simulink model "SNAP_DETUMBLE_barbalatLemma"  (R2024a)
settings: Solver=ode45  StartTime=0.0  StopTime=SNAP_sim_length  FixedStep=0.1  MaxStep=10  MinStep=0.01  RelTol=1e-2  EnableMultiTasking=on
InitFcn:
  | SNAP_Simulink_Init_Function
values from neighbouring files (symbols this model uses):
  bias = [28.8675 28.8675 28.8675]    [SNAP_Simulink_Init_Function.m]    (also in Script_magnetorquer_and_magnetometer.m; SnapParameters.m)
  boira_Imax = boira_max_magnetic_torque./boira_magnetic_gains    [SNAP_Simulink_Init_Function.m]    (also in Script_magnetorquer_and_magnetometer.m; SnapParameters.m)
  boira_magnetic_gains = [2.3 2.3 2.1]    [SNAP_Simulink_Init_Function.m]    (also in Script_magnetorquer_and_magnetometer.m; SnapParameters.m)
  day = C - E + F - floor(30.6001 * G)    [julian2datetime.m]
  EN_2BodyModel = 1    [SNAP_Simulink_Init_Function.m]
  EN_Aero = SNAP_sim_params.aero_enabled    [SNAP_Simulink_Init_Function.m]
  EN_GG = 1    [SNAP_Simulink_Init_Function.m]
  EN_Hyst = 0    [SNAP_Simulink_Init_Function.m]
  EN_Mag = 1    [SNAP_Simulink_Init_Function.m]
  initial_position = SNAP_sim_params.initial_position    [SNAP_Simulink_Init_Function.m]
  initial_velocity = SNAP_sim_params.initial_velocity    [SNAP_Simulink_Init_Function.m]
  lookup_breakpoints_mmeter = linspace(-200,200,50)*10^3    [SNAP_Simulink_Init_Function.m]    (also in Script_magnetorquer_and_magnetometer.m; SnapParameters.m)
  lookup_breakpoints_mtorquer = linspace(-boira_Imax(1)*2,boira_Imax(1)*2,55)    [SNAP_Simulink_Init_Function.m]    (also in Script_magnetorquer_and_magnetometer.m; SnapParameters.m)
  lookup_tabledata_mmeter = lookup_breakpoints_mmeter+max_deviation_mmeter*sin(pi*lookup_breakpoints_mmeter/max_breakpoint_mmeter)    [SNAP_Simulink_Init_Function.m]    (also in Script_magnetorquer_and_magnetometer.m; SnapParameters.m)
  lookup_tabledata_mtorquer = lookup_breakpoints_mtorquer+max_deviation_mtorquer*sin(pi*lookup_breakpoints_mtorquer/max_breakpoint_mtorquer)    [SNAP_Simulink_Init_Function.m]    (also in Script_magnetorquer_and_magnetometer.m; SnapParameters.m)
  noise = 0    [SNAP_Simulink_Init_Function.m]    (also in Script_magnetorquer_and_magnetometer.m; SnapParameters.m)
  noise_variance = 30    [SNAP_Simulink_Init_Function.m]    (also in Script_magnetorquer_and_magnetometer.m; SnapParameters.m)
  rotm_mmeter = eul2rotm([missalingment_x_mmeter missalingment_y_mmeter missalingment_z_mmeter])    [SNAP_Simulink_Init_Function.m]    (also in Script_magnetorquer_and_magnetometer.m; SnapParameters.m)
  rotm_mtorquer = eul2rotm([missalingment_x_mtorquer missalingment_y_mtorquer missalingment_z_mtorquer])    [SNAP_Simulink_Init_Function.m]    (also in Script_magnetorquer_and_magnetometer.m; SnapParameters.m)
  second = (day_fraction - hour - minute / 60) * 3600    [julian2datetime.m]
  SNAP_Br = SNAP_sim_params.Br    [SNAP_Simulink_Init_Function.m]
  SNAP_Bs = SNAP_sim_params.Bs    [SNAP_Simulink_Init_Function.m]
  SNAP_CONST_a3H0 = 7.943e15    (= 7.943e+15)    [SNAP_Simulink_Init_Function.m]
  SNAP_CONST_earth_mag_dipole = [sin(168.6*pi/180)* cos(109.3*pi/180), sin(168.6*pi/180)* sin(109.3*pi/180), cos(168.6*pi/180)]    [SNAP_Simulink_Init_Function.m]
  SNAP_CONST_G_earth = 6.6742e-11    [SNAP_Simulink_Init_Function.m]
  SNAP_CONST_m_earth = 5.9736e24    (= 5.9736e+24)    [SNAP_Simulink_Init_Function.m]
  SNAP_CONST_mu0 = 4*pi*1e-7    (= 1.25663706144e-06)    [SNAP_Simulink_Init_Function.m]
  SNAP_CONST_r_earth = 6.36101e6    (= 6361010)    [SNAP_Simulink_Init_Function.m]
  SNAP_Hc = SNAP_sim_params.Hc    [SNAP_Simulink_Init_Function.m]
  SNAP_init_rates = SNAP_sim_params.init_rates    [SNAP_Simulink_Init_Function.m]
  SNAP_JD = SNAP_sim_params.JD    [SNAP_Simulink_Init_Function.m]
  SNAP_sat_inertia = boira_inertia    [SNAP_Simulink_Init_Function.m]
  SNAP_sat_mass = boira_mass    (= 2)    [SNAP_Simulink_Init_Function.m]
  SNAP_starting_ECI2ECEF_dcm = dcmeci2ecef('IAU-2000/2006',SNAP_sim_params.DateVector)    [SNAP_Simulink_Init_Function.m]
  SNAP_V_hyst = boira_V_hyst    [SNAP_Simulink_Init_Function.m]
undefined symbols (not defined in the file or in its folder): aeroCIP2006, magnitude, SNAPaero
libraries: vrlib x23, simulink x10, sharedtransform x9, aerolibutil x6, aerolibconvert2 x5, aerolibobsolete x1, aerolibanim x1, matrix_library x1
(part 1 of 2)
settings Model: PacingRate=0.010000  Creator=Samir Rawashdeh  LastModifiedBy=pimpao
settings SolverCC: AlgebraicLoopSolver=TrustRegion
settings DataIOCC: SaveFormat=Array  SignalLoggingSaveFormat=ModelDataLogs  ReturnWorkspaceOutputs=off
settings OptimizationCC: ExpressionDepthLimit=2147483647  LifeSpan=inf
settings DebuggingCC: UnderspecifiedInitializationDetection=Classic  MergeDetectMultiDrivingBlocksExec=none  SolverPrmCheckMsg=warning  MultiTaskCondExecSysMsg=warning  MultiTaskRateTransMsg=warning  SingleTaskRateTransMsg=warning  FcnCallInpInsideContextMsg=warning  UnconnectedInputMsg=warning  UnconnectedOutputMsg=warning  UnconnectedLineMsg=warning  StateNameClashWarn=warning  SFUnexpectedBacktrackingDiag=warning  SFNoUnconditionalDefaultTransitionDiag=warning  ArithmeticOperatorsInVariantConditions=warning
settings HardwareCC: ProdBitPerPointer=32  ProdBitPerSizeT=32  ProdBitPerPtrDiffT=32  ProdLargestAtomicFloat=None  ProdIntDivRoundTo=Undefined  ProdEndianess=Unspecified  ProdWordSize=32  ProdHWDeviceType=32-bit Generic
settings ModelReferenceCC: EnableRefExpFcnMdlSchedulingChecks=on  PropagateSignalLabelsOutOfModel=off
settings SFSimCC: SimUseLocalCustomCode=off  CustomCodeUndefinedFunction=UseInterfaceOnly
settings RTWCC: RTWUseLocalCustomCode=off  GPUComputeCapability=3.5
settings CodeAppCC: StateflowObjectComments=on
settings GRTTargetCC: TargetLangStandard=C89/C90 (ANSI)  CombineOutputUpdateFcns=off  GRTInterface=on
settings ConfigComp: CovMetricSettings=dw  CovSaveCumulativeToWorkspaceVar=on  CovSaveSingleToWorkspaceVar=on  CovExternalEMLEnable=off  CovSFcnEnable=off

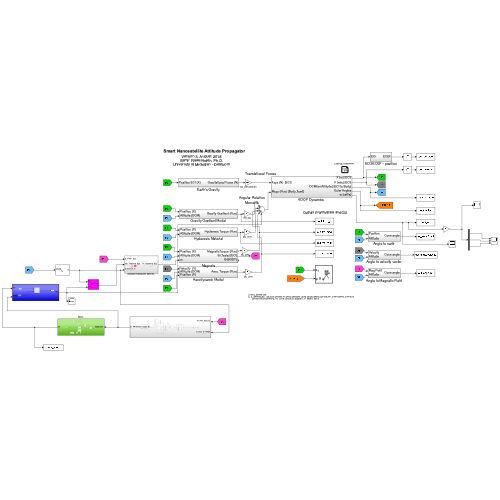
[thumbnail: Simulink's stored preview of the top-level diagram]
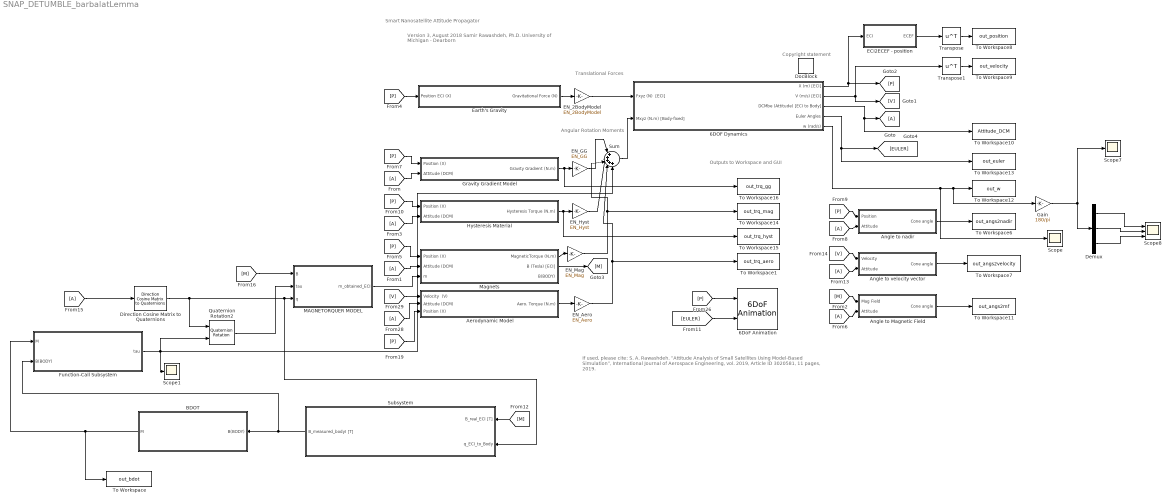
== system SNAP_DETUMBLE_barbalatLemma ==
  note: If used, please cite:
      | S. A. Rawashdeh. “Attitude Analysis of Small Satellites Using Model-Based Simulation”, International Journal of
      |       Aerospace Engineering, vol. 2019, Article ID 3020581, 11 pages, 2019.
  note: Copyright statement
  note: Smart Nanosatellite Attitude Propagator
  note: Version 3, August 2018
      | Samir Rawashdeh, Ph.D.
      | University of Michigan - Dearborn
  note: Translational Forces
  note: Angular Rotation
      | Moments
  note: Outputs to Workspace and GUI
  "6DOF Dynamics " : Subsystem
  6DoF Animation : aerolibanim/6DoF Animation  u1=[-4000 4000 -2000 2000 -5000 -3000]  u2=10  u3=1000000*4  u4=[0 0 0]  u5=Fixed position  u6=[ 1 1 1 ] * 40000000  u7=15  u8=on
  Aerodynamic Model : Subsystem
  Angle to Magnetic Field : Subsystem
  Angle to nadir : Subsystem
  Angle to velocity vector : Subsystem
  BDOT : Subsystem
  Demux : Demux  Outputs=3
  Direction Cosine Matrix to Quaternions : sharedtransform/Direction Cosine Matrix  to Quaternions  aMode=0  action=None  tolerance=eps(2)
      settings: LibrarySourceBlock=|
      | aerolibtransform2/Direction Cosine Matrix
      | to Quaternions
  DocBlock : simulink/Model-Wide Utilities/DocBlock  DocumentType=Text
      content=|
      | % See "help.txt" for documentation. More info in can be found at:
      | % sar-lab.net/snap
      | %
      | % -----------------------------------------------------------------------------
      | %   Copyright (c) 2010-2018 Samir A. Rawashdeh
      | %   Electrical and Computer Engineering
      | %   University of Michigan - Dearborn
      | %
      | %   All rights reserved.
      | %
      | %   Redistribution and use in source and binary forms, with or without
      | %   modification, are permitted provided that the following conditions are
      | %   met:
      | %
      | %       * Redistributions of source code must retain the above copyright
      | %         notice, this list of conditions and the following disclaimer.
      | %       * Redistributions in binary form must reproduce the above copyright
      | %         notice, this list of conditions and the following disclaimer in
      | %         the documentation and/or other materials provided with the distribution
      | %
      | %   THIS SOFTWARE IS PROVIDED BY THE COPYRIGHT HOLDERS AND CONTRIBUTORS "AS IS"
      | %   AND ANY EXPRESS OR IMPLIED WARRANTIES, INCLUDING, BUT NOT LIMITED TO, THE
      | %   IMPLIED WARRANTIES OF MERCHANTABILITY AND FITNESS FOR A PARTICULAR PURPOSE
      | %   ARE DISCLAIMED. IN NO EVENT SHALL THE COPYRIGHT OWNER OR CONTRIBUTORS BE
      | %   LIABLE FOR ANY DIRECT, INDIRECT, INCIDENTAL, SPECIAL, EXEMPLARY, OR
      | %   CONSEQUENTIAL DAMAGES (INCLUDING, BUT NOT LIMITED TO, PROCUREMENT OF
      | %   SUBSTITUTE GOODS OR SERVICES; LOSS OF USE, DATA, OR PROFITS; OR BUSINESS
      | %   INTERRUPTION) HOWEVER CAUSED AND ON ANY THEORY OF LIABILITY, WHETHER IN
      | %   CONTRACT, STRICT LIABILITY, OR TORT (INCLUDING NEGLIGENCE OR OTHERWISE)
      | %   ARISING IN ANY WAY OUT OF THE USE OF THIS SOFTWARE, EVEN IF ADVISED OF THE
      | %   POSSIBILITY OF SUCH DAMAGE.
      | %
      | % ----------------------------------------------------------------------------
  ECI2ECEF - position : Subsystem
  EN_2BodyModel : Gain  Gain=EN_2BodyModel
  "EN_Aero " : Gain  Gain=EN_Aero
  EN_GG : Gain  Gain=EN_GG
  EN_Hyst : Gain  Gain=EN_Hyst
  EN_Mag : Gain  Gain=EN_Mag
  Earth's Gravity : Subsystem
  From{,1,3,6,8,13,15,28} (8 alike) : From
      From settings: CloseFcn=tagdialog Close
      From1 settings: CloseFcn=tagdialog Close
      From13 settings: CloseFcn=tagdialog Close
      From28 settings: CloseFcn=tagdialog Close
      From3 settings: CloseFcn=tagdialog Close
      From6 settings: CloseFcn=tagdialog Close
      From8 settings: CloseFcn=tagdialog Close
  Function-Call Subsystem : Subsystem  TreatAsAtomicUnit=on
  Gain : Gain  Gain=180/pi
  Goto : Goto
  Gravity Gradient Model : Subsystem
  Hysteresis Material : Subsystem
  MAGNETORQUER MODEL : Subsystem
  Magnets : Subsystem
  Quaternion Rotation2 : aerolibutil/Quaternion Rotation
  Scope : Scope
  Scope1 : Scope
  Scope7 : Scope
  Scope8 : Scope  NumInputPorts=3
  Subsystem : Subsystem
  Sum : Sum  Inputs=|+++++
  To Workspace : ToWorkspace  VariableName=out_bdot  SaveFormat=Structure With Time  SampleTime=-1
  To Workspace1 : ToWorkspace  VariableName=out_trq_aero  SaveFormat=Structure With Time  SampleTime=-1
  To Workspace10 : ToWorkspace  VariableName=Attitude_DCM  SaveFormat=Structure With Time  SampleTime=-1
  To Workspace11 : ToWorkspace  VariableName=out_angs2mf  SaveFormat=Structure With Time  SampleTime=-1
  To Workspace12 : ToWorkspace  VariableName=out_w  SaveFormat=Structure With Time  SampleTime=-1
  To Workspace13 : ToWorkspace  VariableName=out_euler  SaveFormat=Structure With Time  SampleTime=-1
  To Workspace14 : ToWorkspace  VariableName=out_trq_mag  SaveFormat=Structure With Time  SampleTime=-1
  To Workspace15 : ToWorkspace  VariableName=out_trq_hyst  SaveFormat=Structure With Time  SampleTime=-1
  To Workspace16 : ToWorkspace  VariableName=out_trq_gg  SaveFormat=Structure With Time  SampleTime=-1
  To Workspace6 : ToWorkspace  VariableName=out_angs2nadir  SaveFormat=Structure With Time  SampleTime=-1
  To Workspace7 : ToWorkspace  VariableName=out_angs2velocity  SaveFormat=Structure With Time  SampleTime=-1
  To Workspace8 : ToWorkspace  VariableName=out_position  SaveFormat=Structure With Time  SampleTime=-1
  To Workspace9 : ToWorkspace  VariableName=out_velocity  SaveFormat=Structure With Time  SampleTime=-1
  Transpose : Math  Operator=transpose  SignedPower=on
  Transpose1 : Math  Operator=transpose  SignedPower=on
  wires:
  Transpose/1 -> To Workspace8/1
  Transpose1/1 -> To Workspace9/1
  "6DOF Dynamics "/3(DCMbe (Attitude) [ECI to Body]) -> To Workspace10/1, Goto/1
  "6DOF Dynamics "/4(Euler Angles) -> [EULER], To Workspace13/1
  "6DOF Dynamics "/5(w (rad/s)) -> Scope/1, Gain/1, To Workspace12/1
  Gravity Gradient Model/1(Gravity Gradient (N.m)) -> To Workspace16/1, EN_GG/1
  Hysteresis Material/1(Hysteresis Torque (N.m)) -> EN_Hyst/1, To Workspace15/1
  EN_Mag/1 -> Sum/3, To Workspace14/1
  Angle to nadir/1(Cone angle) -> To Workspace6/1
  Angle to velocity vector/1(Cone angle) -> To Workspace7/1
  [P] -> Earth's Gravity/1(Position ECI (X))
  "6DOF Dynamics "/1(X (m) [ECI]) -> ECI2ECEF - position/1(ECI), [P]
  "6DOF Dynamics "/2(V (m/s) [ECI]) -> Transpose1/1, [V]
  [P] -> Gravity Gradient Model/1(Position (X))
  From/1 -> Gravity Gradient Model/2(Attitude (DCM))
  [P] -> Magnets/1(Position (X))
  From1/1 -> Magnets/2(Attitude (DCM))
  Magnets/1(MagneticTorque (N.m)) -> EN_Mag/1
  From8/1 -> Angle to nadir/2(Attitude)
  [P] -> Angle to nadir/1(Position)
  From13/1 -> Angle to velocity vector/2(Attitude)
  [V] -> Angle to velocity vector/1(Velocity)
  ECI2ECEF - position/1(ECEF) -> Transpose/1
  Magnets/2(B (Tesla) [ECI]) -> [M]
  Earth's Gravity/1(Gravitational Force (N)) -> EN_2BodyModel/1
  From6/1 -> Angle to Magnetic Field/2(Attitude)
  Angle to Magnetic Field/1(Cone angle) -> To Workspace11/1
  [M] -> Angle to Magnetic Field/1(Mag Field)
  EN_GG/1 -> Sum/1
  EN_Hyst/1 -> Sum/2
  [V] -> Aerodynamic Model/1(Velocity  (V))
  From28/1 -> Aerodynamic Model/2(Attitude (DCM))
  [P] -> Aerodynamic Model/3(Position (X))
  [P] -> 6DoF Animation/1
  EN_2BodyModel/1 -> "6DOF Dynamics "/1(Fxyz (N)  [ECI])
  Sum/1 -> "6DOF Dynamics "/2(Mxyz (N.m) [Body-fixed])
  [P] -> Hysteresis Material/1(Position (X))
  From3/1 -> Hysteresis Material/2(Attitude (DCM))
  Aerodynamic Model/1(Aero. Torque (N.m)) -> "EN_Aero "/1
  "EN_Aero "/1 -> Sum/4, To Workspace1/1
  [EULER] -> 6DoF Animation/2
  Gain/1 -> Scope7/1, Demux/1
  Demux/1 -> Scope8/1
  Demux/2 -> Scope8/2
  Demux/3 -> Scope8/3
  MAGNETORQUER MODEL/1(m_obtained_ECI) -> Magnets/3(m)
  Direction Cosine Matrix to Quaternions/1 -> Quaternion Rotation2/1, MAGNETORQUER MODEL/3(q), Subsystem/2(q_ECI_to_Body)
  [M] -> MAGNETORQUER MODEL/1(B)
  Function-Call Subsystem/1(tau) -> Quaternion Rotation2/2, Sum/5, Scope1/1
  Quaternion Rotation2/1 -> MAGNETORQUER MODEL/2(tau)
  BDOT/1(M) -> To Workspace/1, Function-Call Subsystem/1(M)
  Subsystem/1(B_measured_bodyI [T]) -> Function-Call Subsystem/2(B(BODY)), BDOT/1(B(BODY))
  [M] -> Subsystem/1(B_real_ECI [T])
  From15/1 -> Direction Cosine Matrix to Quaternions/1

== system SNAP_DETUMBLE_barbalatLemma/6DOF Dynamics  ==
  Fxyz (N)  [ECI] : Inport
  Mxyz (N.m) [Body-fixed] : Inport  Port=2
  Rotations - 6DoF (Quaternion) : aerolibobsolete/6DoF (Euler Angles)  units=Metric (MKS)  mtype=Fixed  rep=Quaternion  xme_0=[0 0 0] % not used  Vm_0=[0 0 0] % not used  eul_0=[0 0 0] %[0 pi/1.1 0]  pm_0=SNAP_init_rates %(ones(1,3)*0.5-rand(1,3) )* 2 * .3 *pi/180;  mass_0=SNAP_sat_mass  mass_e=0  mass_f=0  inertia=SNAP_sat_inertia  inertia_e=eye(3)  inertia_f=eye(3)  k_quat=1.0
  Terminator{,1..3,5} (5 alike) : Terminator
  Translation : Subsystem
  zero : Constant  Value=[0 0 0]
  X (m) [ECI] : Outport
  V (m/s) [ECI] : Outport  Port=2
  DCMbe (Attitude) [ECI to Body] : Outport  Port=3
  Euler Angles : Outport  Port=4
  w (rad/s) : Outport  Port=5
  wires:
  Rotations - 6DoF (Quaternion)/2 -> Terminator/1
  Rotations - 6DoF (Quaternion)/1 -> Terminator2/1
  Rotations - 6DoF (Quaternion)/5 -> Terminator1/1
  Translation/1(Xe(m) (ECI)) -> X (m) [ECI]/1
  Translation/2(Ve(m/s) (ECI)) -> V (m/s) [ECI]/1
  Rotations - 6DoF (Quaternion)/6 -> w (rad/s)/1
  Rotations - 6DoF (Quaternion)/8 -> Terminator5/1
  Rotations - 6DoF (Quaternion)/7 -> Terminator3/1
  zero/1 -> Rotations - 6DoF (Quaternion)/1
  Fxyz (N)  [ECI]/1 -> Translation/1(Fxyz (N) (inECI))
  Mxyz (N.m) [Body-fixed]/1 -> Rotations - 6DoF (Quaternion)/2
  Rotations - 6DoF (Quaternion)/3 -> Euler Angles/1
  Rotations - 6DoF (Quaternion)/4 -> DCMbe (Attitude) [ECI to Body]/1

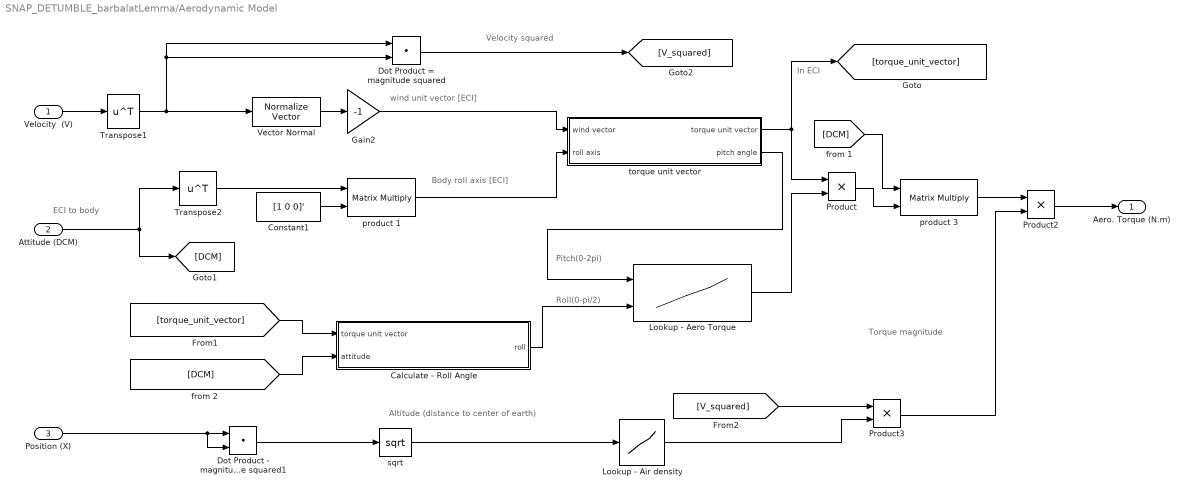
== system SNAP_DETUMBLE_barbalatLemma/Aerodynamic Model ==
  note: Pitch(0-2pi)
  note: wind unit vector [ECI]
  note: Torque magnitude
  note: Body roll axis [ECI]
  note: In ECI
  note: ECI to body
  note: Velocity squared
  note: Roll(0-pi/2)
  note: Altitude (distance to center of earth)
  Velocity  (V) : Inport
  Attitude (DCM) : Inport  Port=2
  Position (X) : Inport  Port=3
  Calculate - Roll Angle : Subsystem
  Constant1 : Constant  Value=[1 0 0]'
  Dot Product - magnitude squared1 : DotProduct  OutDataTypeStr=Inherit: Inherit via internal rule
  Dot Product = magnitude squared : DotProduct  OutDataTypeStr=Inherit: Inherit via internal rule
  Gain2 : Gain  Gain=-1
  Lookup - Aero Torque : Lookup2D  RowIndex=SNAPaero.pitch  ColumnIndex=SNAPaero.roll  Table=SNAPaero.T  SaturateOnIntegerOverflow=off  InputSameDT=off
  Lookup - Air density : Lookup  InputValues=SNAPaero.alt_range*1000 + SNAP_CONST_r_earth  Table=SNAPaero.av_density_vs_alt  SaturateOnIntegerOverflow=off
  Product : Product  RndMeth=Zero
  Product2 : Product  RndMeth=Zero
  Product3 : Product  RndMeth=Zero
  Transpose1 : Math  Operator=transpose  SignedPower=on
  Transpose2 : Math  Operator=transpose  SignedPower=on
  Vector Normal : vrlib/Utilities/Normalize Vector  maxzero=0
  product 1 : Product  Multiplication=Matrix(*)  RndMeth=Zero
  product 3 : Product  Multiplication=Matrix(*)  RndMeth=Zero
  sqrt : Math  Operator=sqrt  SignedPower=on
  torque unit vector : Subsystem
  Aero. Torque (N.m) : Outport
  wires:
  Velocity  (V)/1 -> Transpose1/1
  Dot Product = magnitude squared/1 -> [V_squared]
  Vector Normal/1 -> Gain2/1
  Gain2/1 -> torque unit vector/1(wind vector)
  product 1/1 -> torque unit vector/2(roll axis)
  torque unit vector/1(torque unit vector) -> Product/1, [torque_unit_vector]
  Lookup - Aero Torque/1 -> Product/2
  [DCM] -> product 3/1
  Transpose1/1 -> Vector Normal/1, Dot Product = magnitude squared/2, Dot Product = magnitude squared/1
  Constant1/1 -> product 1/2
  Attitude (DCM)/1 -> [DCM], Transpose2/1
  Product/1 -> product 3/2
  Calculate - Roll Angle/1(roll) -> Lookup - Aero Torque/2
  torque unit vector/2(pitch angle) -> Lookup - Aero Torque/1
  Transpose2/1 -> product 1/1
  [torque_unit_vector] -> Calculate - Roll Angle/1(torque unit vector)
  [DCM] -> Calculate - Roll Angle/2(attitude)
  Position (X)/1 -> Dot Product - magnitude squared1/1, Dot Product - magnitude squared1/2
  Dot Product - magnitude squared1/1 -> sqrt/1
  sqrt/1 -> Lookup - Air density/1
  Lookup - Air density/1 -> Product3/2
  Product3/1 -> Product2/2
  [V_squared] -> Product3/1
  Product2/1 -> Aero. Torque (N.m)/1
  product 3/1 -> Product2/1

== system SNAP_DETUMBLE_barbalatLemma/Angle to Magnetic Field ==
  note: velocity vector
  Mag Field : Inport
  Attitude : Inport  Port=2
  Normalize Vector : vrlib/Utilities/Normalize Vector  maxzero=0
  cosines to body axes : Subsystem
  Cone angle : Outport
  wires:
  Mag Field/1 -> Normalize Vector/1
  Attitude/1 -> cosines to body axes/2(Attitude)
  cosines to body axes/1(Cone Angles) -> Cone angle/1
  Normalize Vector/1 -> cosines to body axes/1(Reference Vector)

== system SNAP_DETUMBLE_barbalatLemma/Angle to nadir ==
  note: vector from satellite to earth (nadir)
  Position : Inport
  Attitude : Inport  Port=2
  Gain2 : Gain  Gain=-1
  Normalize Vector : vrlib/Utilities/Normalize Vector  maxzero=0
  cosines to body axes : Subsystem
  Cone angle : Outport
  wires:
  Normalize Vector/1 -> Gain2/1
  Position/1 -> Normalize Vector/1
  cosines to body axes/1(Cone Angles) -> Cone angle/1
  Gain2/1 -> cosines to body axes/1(Reference Vector)
  Attitude/1 -> cosines to body axes/2(Attitude)

== system SNAP_DETUMBLE_barbalatLemma/Angle to velocity vector ==
  note: velocity vector
  Velocity : Inport
  Attitude : Inport  Port=2
  Normalize Vector : vrlib/Utilities/Normalize Vector  maxzero=0
  cosines to body axes : Subsystem
  Cone angle : Outport
  wires:
  Velocity/1 -> Normalize Vector/1
  Attitude/1 -> cosines to body axes/2(Attitude)
  cosines to body axes/1(Cone Angles) -> Cone angle/1
  Normalize Vector/1 -> cosines to body axes/1(Reference Vector)

== system SNAP_DETUMBLE_barbalatLemma/BDOT ==
  B(BODY) : Inport
  Constant1 : Constant  Value=[0.6,0,0;0,0.5,0;0,0,0.4]
  Discrete Derivative1 : simulink/Discrete/Discrete Derivative  gainval=1.0  ICPrevScaledInput=0.0  OutMin=[]  OutMax=[]  OutDataType=fixdt(1, 16)  OutScaling=2^-10  DoSatur=off
  Gain1 : Gain  Gain=-1
  MATLAB Function : MATLAB Function  TreatAsAtomicUnit=on
  Matrix Divide : Product  Inputs=*/  Multiplication=Matrix(*)
  MatrixMultiply : Product  Multiplication=Matrix(*)
  Normalize Vector : vrlib/Utilities/Normalize Vector  maxzero=0
  Square : Math  Operator=square
  Terminator : Terminator
  M : Outport
  wires:
  B(BODY)/1 -> Discrete Derivative1/1, Normalize Vector/1, MATLAB Function/1(u)
  MATLAB Function/1(y) -> Matrix Divide/2
  MatrixMultiply/1 -> Matrix Divide/1
  Gain1/1 -> MatrixMultiply/1
  Normalize Vector/1 -> Square/1
  Matrix Divide/1 -> M/1
  Square/1 -> Terminator/1
  Constant1/1 -> Gain1/1
  Discrete Derivative1/1 -> MatrixMultiply/2

== system SNAP_DETUMBLE_barbalatLemma/ECI2ECEF - position ==
  ECI : Inport
  Constant : Constant  Value=[0 0]
  Constant1 : Constant  Commented=on  Value=SNAP_JD
  Constant2 : Constant  Value=SNAP_starting_ECI2ECEF_dcm
  Direction Cosine Matrix ECI to ECEF1 : Subsystem  Commented=on  AncestorBlock=aerolibtransform2/Direction Cosine Matrix ECI to ECEF  mask{red=IAU-2000/2006, deltaT=Sec, errorflag=Error, extraparamflag=off}
      mask prompts: red "aeroblks:aeroblktransform:blockDCMECItoECEFParamReduction"; deltaT "aeroblks:aeroblktransform:blockDCMECItoECEFParamTimeincrement"; errorflag "aeroblks:aeroblktransform:blockDCMECItoECEFParamActionforoutofrangeinput"; extraparamflag "aeroblks:aeroblktransform:blockDCMECItoECEFParamHigheraccuracyparameters"
      settings: AttributesFormatString=%<red>
      mask TypeOptions red: aeroblks:aeroblktransform:blockDCMECItoECEFParamComboIAU76FK5 | aeroblks:aeroblktransform:blockDCMECItoECEFParamComboIAU20002006
      mask TypeOptions deltaT: aeroblks:aeroblktransform:blockDCMECItoECEFParamComboNone | aeroblks:aeroblktransform:blockDCMECItoECEFParamComboDay | aeroblks:aeroblktransform:blockDCMECItoECEFParamComboHour | aeroblks:aeroblktransform:blockDCMECItoECEFParamComboMin | aeroblks:aeroblktransform:blockDCMECItoECEFParamComboSec
      mask TypeOptions errorflag: aeroblks:aeroblktransform:blockDCMECItoECEFParamComboNone | aeroblks:aeroblktransform:blockDCMECItoECEFParamComboWarning | aeroblks:aeroblktransform:blockDCMECItoECEFParamComboError
      mask Display:
      | port_label('output',1,'DCM_{fi}','texmode','on')
      | port_label('input',1,'JD')
  Gain : Gain  Gain=-1
  Mux : Mux  Inputs=2
  Ramp1 : simulink/Sources/Ramp  slope="7.292115856e-5   %2*pi/(24*60*60)  %radians/second (one rotation per day )"  start=0  InitialOutput=0
  Rotation Angles to Direction Cosine Matrix : sharedtransform/Rotation Angles to Direction Cosine Matrix  rotationOrder=ZYX  aMode=aMode
  product 1 : Product  Multiplication=Matrix(*)  RndMeth=Zero
  product 2 : Product  Multiplication=Matrix(*)  RndMeth=Zero
  ECEF : Outport
  wires:
  product 2/1 -> ECEF/1
  ECI/1 -> product 2/1
  Constant1/1 -> Direction Cosine Matrix ECI to ECEF1/1(JD)
  Ramp1/1 -> Gain/1
  Gain/1 -> Mux/1
  Mux/1 -> Rotation Angles to Direction Cosine Matrix/1
  Constant/1 -> Mux/2
  product 1/1 -> product 2/2
  Rotation Angles to Direction Cosine Matrix/1 -> product 1/2
  Constant2/1 -> product 1/1

== system SNAP_DETUMBLE_barbalatLemma/Earth's Gravity ==
  note: Gravitational
      | acceleration vector
  note: magnitude of acceleration due to gravity
  note: Unit vector towards Nadir
  note: a_gravity = G*m/r^2
  Position ECI (X) : Inport
  Constant : Constant  Value=SNAP_CONST_r_earth
  Divide : Product  Inputs=*/
  Gain1 : Gain  Gain=-1
  Gain2 : Gain  Gain=SNAP_sat_mass
  Gravitational Constant : Constant  Value=SNAP_CONST_m_earth*SNAP_CONST_G_earth
  Math Function : Math  Operator=sqrt  SignedPower=on
  Product : Product  RndMeth=Zero
  Scope4 : Scope
  Sum : Sum  Inputs=|+-
  Vector Dot Product = magnitude squared : DotProduct  OutDataTypeStr=Inherit: Inherit via internal rule
  Vector Normal : vrlib/Utilities/Normalize Vector  maxzero=0
  Gravitational Force (N) : Outport
  wires:
  Position ECI (X)/1 -> Vector Normal/1, Vector Dot Product = magnitude squared/1, Vector Dot Product = magnitude squared/2
  Vector Normal/1 -> Gain1/1
  Gain1/1 -> Product/1
  Product/1 -> Gain2/1
  Vector Dot Product = magnitude squared/1 -> Divide/2, Math Function/1
  Divide/1 -> Product/2
  Gravitational Constant/1 -> Divide/1
  Gain2/1 -> Gravitational Force (N)/1
  Math Function/1 -> Sum/1
  Sum/1 -> Scope4/1
  Constant/1 -> Sum/2

== system SNAP_DETUMBLE_barbalatLemma/Function-Call Subsystem ==
  M : Inport
  B(BODY) : Inport  Port=2
  Cross Product : matrix_library/Cross Product
  tau : Outport
  wires:
  M/1 -> Cross Product/1
  B(BODY)/1 -> Cross Product/2
  Cross Product/1 -> tau/1

== system SNAP_DETUMBLE_barbalatLemma/Gravity Gradient Model ==
  note: (3*mu/Rs^4*) * Rs = (3*mu/Rs^3) * rs
  note: Nadir [body]
  note: position of satellite [ECI]
  note: Nadir unit vector
      | [body]
  note: Anti-nadir [body]
  note: r^4
  Position (X) : Inport
  Attitude (DCM) : Inport  Port=2
  Constant : Constant  Value=3*SNAP_CONST_m_earth*SNAP_CONST_G_earth
  Constant1 : Constant  Value=SNAP_sat_inertia
  Cross Product : vrlib/Utilities/Cross Product
  Divide : Product  Inputs=*/
  Dot Product = magnitude squared : DotProduct  OutDataTypeStr=Inherit: Inherit via internal rule
  Gain : Gain  Gain=-1
  Gain1 : Gain  Gain=-1
  Math Function : Math  Operator=square  SignedPower=on
  Math Function1 : Math  Operator=transpose  SignedPower=on
  Product (not cross) : Product  RndMeth=Zero
  Vector Normal : vrlib/Utilities/Normalize Vector  maxzero=0
  product 1 : Product  Multiplication=Matrix(*)  RndMeth=Zero
  product 2 : Product  Multiplication=Matrix(*)  RndMeth=Zero
  Gravity Gradient (N.m) : Outport
  wires:
  Product (not cross)/1 -> Cross Product/1
  Divide/1 -> Product (not cross)/2
  Constant/1 -> Divide/1
  Math Function/1 -> Divide/2
  Vector Normal/1 -> Gain/1
  Cross Product/1 -> Gravity Gradient (N.m)/1
  Dot Product = magnitude squared/1 -> Math Function/1
  Gain/1 -> product 2/2
  product 2/1 -> Cross Product/2
  Constant1/1 -> product 2/1
  Position (X)/1 -> Dot Product = magnitude squared/2, Dot Product = magnitude squared/1, Math Function1/1
  Attitude (DCM)/1 -> product 1/1
  product 1/1 -> Vector Normal/1, Gain1/1
  Gain1/1 -> Product (not cross)/1
  Math Function1/1 -> product 1/2

== system SNAP_DETUMBLE_barbalatLemma/Hysteresis Material ==
  note: ECI to Body
  note: T = m X B
  note: B_earth
  note: B_earth [body]
  note: m [body]
  Position (X) : Inport
  Attitude (DCM) : Inport  Port=2
  Cross Product : vrlib/Utilities/Cross Product
  Eearth L-Shell Magnetic Model : Subsystem
  Gain : Gain  Gain=1/SNAP_CONST_mu0
  Hysteresis Curve Model : Subsystem
  Product : Product  Multiplication=Matrix(*)  RndMeth=Zero
  Transpose : Math  Operator=transpose  SignedPower=on
  m = B*V/mu0 : Product  RndMeth=Zero
  zero : Constant  Value=SNAP_V_hyst/SNAP_CONST_mu0
  Hysteresis Torque (N.m) : Outport
  wires:
  Product/1 -> Gain/1, Cross Product/2
  Cross Product/1 -> Hysteresis Torque (N.m)/1
  zero/1 -> m = B*V/mu0/2
  m = B*V/mu0/1 -> Cross Product/1
  Attitude (DCM)/1 -> Product/1
  Eearth L-Shell Magnetic Model/1(B (Tesla) in ECI) -> Transpose/1
  Transpose/1 -> Product/2
  Gain/1 -> Hysteresis Curve Model/1(H)
  Hysteresis Curve Model/1(B) -> m = B*V/mu0/1
  Position (X)/1 -> Eearth L-Shell Magnetic Model/1(Position in ECI)

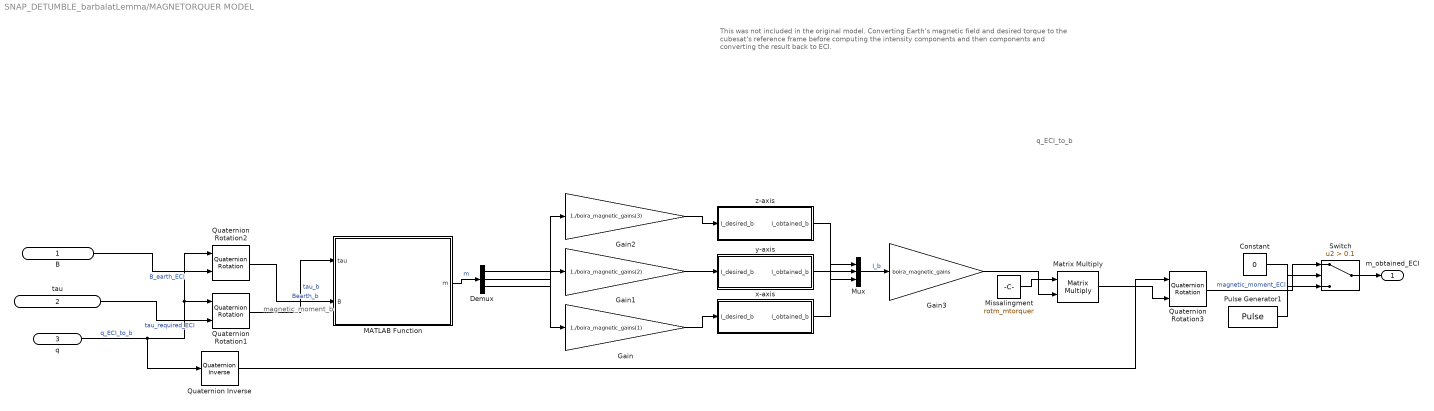
== system SNAP_DETUMBLE_barbalatLemma/MAGNETORQUER MODEL ==
  note: magnetic_moment_b
  note: This was not included in the original model.
      | Converting Earth's magnetic field and desired torque to the cubesat's reference frame before computing the intensity components and then  components and converting the result back to ECI.
  note: q_ECI_to_b
  B : Inport
  tau : Inport  Port=2
  q : Inport  Port=3
  Constant : Constant  Value=0
  Demux : Demux  Outputs=3
  Gain : Gain  Gain=1./boira_magnetic_gains(1)
  Gain1 : Gain  Gain=1./boira_magnetic_gains(2)
  Gain2 : Gain  Gain=1./boira_magnetic_gains(3)
  Gain3 : Gain  Gain=boira_magnetic_gains
  MATLAB Function : MATLAB Function  TreatAsAtomicUnit=on
  Matrix Multiply : Product  Multiplication=Matrix(*)
  Missalingment : Constant  Value=rotm_mtorquer  OutDataTypeStr=Inherit: Inherit via back propagation
  Mux : Mux  Inputs=3
  Pulse Generator1 : DiscretePulseGenerator  PulseType=Time based  Period=1  PulseWidth=80  PhaseDelay=0.2
  Quaternion Inverse : aerolibutil/Quaternion Inverse
  Quaternion Rotation1 : aerolibutil/Quaternion Rotation
  Quaternion Rotation2 : aerolibutil/Quaternion Rotation
  Quaternion Rotation3 : aerolibutil/Quaternion Rotation
  Switch : Switch  Criteria=u2 > Threshold  Threshold=0.1  SaturateOnIntegerOverflow=off  InputSameDT=off
  x-axis : Subsystem
  y-axis : Subsystem
  z-axis : Subsystem
  m_obtained_ECI : Outport
  wires:
  tau/1 -> Quaternion Rotation1/2  "tau_required_ECI"
  Gain1/1 -> y-axis/1(I_desired_b)
  Demux/1 -> Gain/1
  Quaternion Rotation3/1 -> Switch/1  "magnetic_moment_ECI"
  Gain3/1 -> Matrix Multiply/2
  Pulse Generator1/1 -> Switch/2
  MATLAB Function/1(m) -> Demux/1  "m"
  B/1 -> Quaternion Rotation2/2  "B_earth_ECI"
  Demux/3 -> Gain2/1
  Gain/1 -> x-axis/1(I_desired_b)
  Switch/1 -> m_obtained_ECI/1
  x-axis/1(I_obtained_b) -> Mux/1
  z-axis/1(I_obtained_b) -> Mux/3
  q/1 -> Quaternion Rotation2/1, Quaternion Rotation1/1, Quaternion Inverse/1  "q_ECI_to_b"
  y-axis/1(I_obtained_b) -> Mux/2
  Constant/1 -> Switch/3
  Quaternion Rotation1/1 -> MATLAB Function/1(tau)  "tau_b"
  Mux/1 -> Gain3/1  "I_b"
  Quaternion Inverse/1 -> Quaternion Rotation3/1
  Missalingment/1 -> Matrix Multiply/1
  Demux/2 -> Gain1/1
  Matrix Multiply/1 -> Quaternion Rotation3/2
  Quaternion Rotation2/1 -> MATLAB Function/2(B)  "Bearth_b"
  Gain2/1 -> z-axis/1(I_desired_b)

== system SNAP_DETUMBLE_barbalatLemma/Magnets ==
  note: T = m X B
  note: B_earth [body]
  note: ECI to Body
  Position (X) : Inport
  Attitude (DCM) : Inport  Port=2
  m : Inport  Port=3
  Cross Product : vrlib/Utilities/Cross Product
  Eearth L-Shell Magnetic Model : Subsystem
  Product : Product  Multiplication=Matrix(*)  RndMeth=Zero
  Transpose : Math  Operator=transpose  SignedPower=on
  MagneticTorque (N.m) : Outport
  B (Tesla) [ECI] : Outport  Port=2
  B(BODY) : Outport  Port=3
  wires:
  Position (X)/1 -> Eearth L-Shell Magnetic Model/1(Position in ECI)
  Product/1 -> B(BODY)/1, Cross Product/2
  Cross Product/1 -> MagneticTorque (N.m)/1
  m/1 -> Cross Product/1
  Attitude (DCM)/1 -> Product/1
  Eearth L-Shell Magnetic Model/1(B (Tesla) in ECI) -> Transpose/1, B (Tesla) [ECI]/1
  Transpose/1 -> Product/2

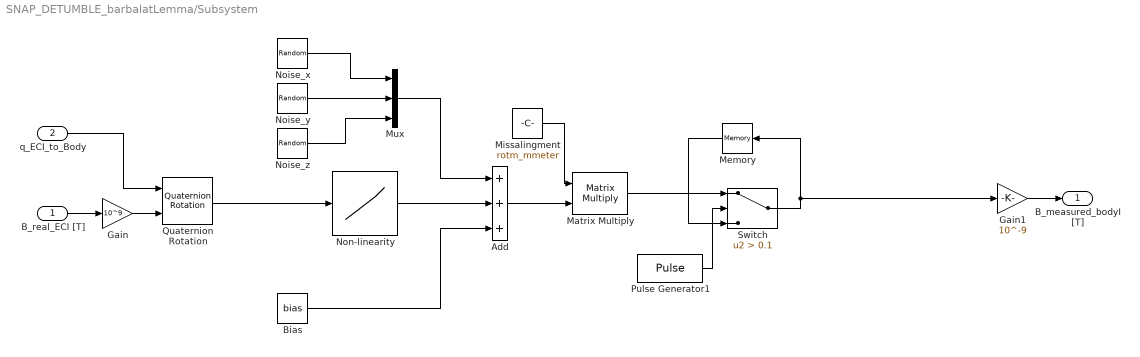
== system SNAP_DETUMBLE_barbalatLemma/Subsystem ==
  B_real_ECI [T] : Inport
  q_ECI_to_Body : Inport  Port=2
  Add : Sum  Inputs=+++
  Bias : Constant  Value=bias
  Gain : Gain  Gain=10^9
  Gain1 : Gain  Gain=10^-9
  Matrix Multiply : Product  Multiplication=Matrix(*)
  Memory : Memory
  Missalingment : Constant  Value=rotm_mmeter  OutDataTypeStr=Inherit: Inherit via back propagation
  Mux : Mux  Inputs=3
  Noise_x : RandomNumber  Mean=noise  Variance=noise_variance  Seed=rand(1,1)*100000  SampleTime=0.1
  Noise_y : RandomNumber  Mean=noise  Variance=noise_variance  Seed=rand(1,1)*100000  SampleTime=0.1
  Noise_z : RandomNumber  Mean=noise  Variance=noise_variance  Seed=rand(1,1)*100000  SampleTime=0.1
  Non-linearity : Lookup_n-D  NumberOfTableDimensions=1  BreakpointsForDimension1=lookup_breakpoints_mmeter  Table=lookup_tabledata_mmeter  InternalRulePriority=Speed  RndMeth=Simplest
  Pulse Generator1 : DiscretePulseGenerator  PulseType=Time based  Period=1  PulseWidth=20
  Quaternion Rotation : aerolibutil/Quaternion Rotation
  Switch : Switch  Criteria=u2 > Threshold  Threshold=0.1  SaturateOnIntegerOverflow=off  InputSameDT=off
  B_measured_bodyI [T] : Outport
  wires:
  Noise_x/1 -> Mux/1
  Pulse Generator1/1 -> Switch/2
  Missalingment/1 -> Matrix Multiply/1
  Gain1/1 -> B_measured_bodyI [T]/1
  q_ECI_to_Body/1 -> Quaternion Rotation/1
  Matrix Multiply/1 -> Switch/1
  Non-linearity/1 -> Add/2
  Quaternion Rotation/1 -> Non-linearity/1
  Bias/1 -> Add/3
  Memory/1 -> Switch/3
  Switch/1 -> Gain1/1, Memory/1
  Noise_y/1 -> Mux/2
  Mux/1 -> Add/1
  Add/1 -> Matrix Multiply/2
  B_real_ECI [T]/1 -> Gain/1
  Gain/1 -> Quaternion Rotation/2
  Noise_z/1 -> Mux/3

== system SNAP_DETUMBLE_barbalatLemma/6DOF Dynamics /Translation ==
  note: Force
  note: Acceleration
  note: Velocity
  note: Position
  Fxyz (N) (inECI) : Inport
  Gain : Gain  Gain=1/SNAP_sat_mass
  Integrator : Integrator  InitialCondition=initial_velocity
  Integrator1 : Integrator  InitialCondition=initial_position
  Xe(m) (ECI) : Outport
  Ve(m/s) (ECI) : Outport  Port=2
  wires:
  Fxyz (N) (inECI)/1 -> Gain/1
  Gain/1 -> Integrator/1
  Integrator/1 -> Integrator1/1, Ve(m/s) (ECI)/1
  Integrator1/1 -> Xe(m) (ECI)/1

== system SNAP_DETUMBLE_barbalatLemma/Aerodynamic Model/Calculate - Roll Angle ==
  note: pitch axis in ECI
  note: Roll(0-pi/2)
  torque unit vector : Inport
  attitude : Inport  Port=2
  Constant2 : Constant  Value=[0 1 0]'
  Constant3 : Constant  Value=pi/2
  Dot Product : DotProduct  OutDataTypeStr=Inherit: Inherit via internal rule
  Modulus : Math  Operator=mod  SignedPower=on
  Trigonometric Function1 : Trigonometry  Operator=acos
  product 2 : Product  Multiplication=Matrix(*)  RndMeth=Zero
  roll : Outport
  wires:
  torque unit vector/1 -> Dot Product/1
  product 2/1 -> Dot Product/2
  Dot Product/1 -> Trigonometric Function1/1
  Trigonometric Function1/1 -> Modulus/1
  Constant3/1 -> Modulus/2
  Modulus/1 -> roll/1
  Constant2/1 -> product 2/2
  attitude/1 -> product 2/1

== system SNAP_DETUMBLE_barbalatLemma/Aerodynamic Model/torque unit vector ==
  wind vector : Inport
  roll axis : Inport  Port=2
  Cross Product : vrlib/Utilities/Cross Product
  Dot Product : DotProduct  OutDataTypeStr=Inherit: Inherit via internal rule
  Normalize Vector : vrlib/Utilities/Normalize Vector  maxzero=0
  Trigonometric Function2 : Trigonometry  Operator=acos
  torque unit vector : Outport
  pitch angle : Outport  Port=2
  wires:
  Normalize Vector/1 -> torque unit vector/1
  Cross Product/1 -> Normalize Vector/1
  wind vector/1 -> Cross Product/1, Dot Product/1
  roll axis/1 -> Cross Product/2, Dot Product/2
  Dot Product/1 -> Trigonometric Function2/1
  Trigonometric Function2/1 -> pitch angle/1

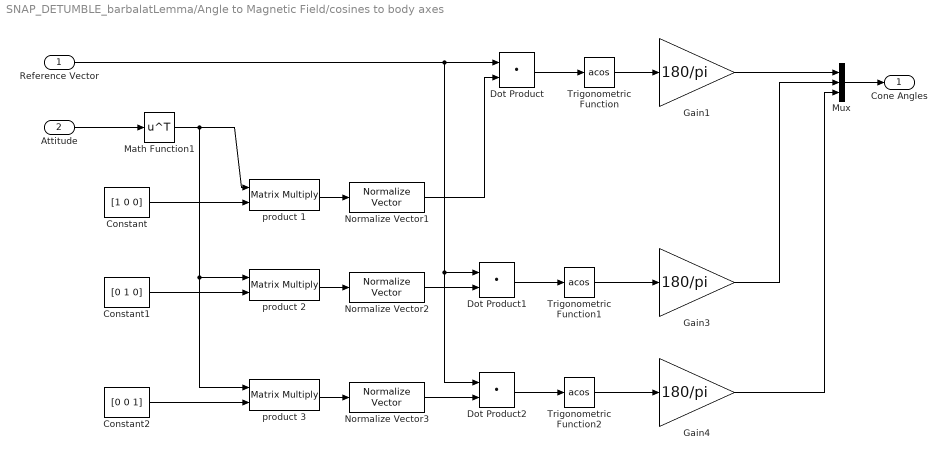
== system SNAP_DETUMBLE_barbalatLemma/Angle to Magnetic Field/cosines to body axes ==
  Reference Vector : Inport
  Attitude : Inport  Port=2
  Constant : Constant  Value=[1 0 0]
  Constant1 : Constant  Value=[0 1 0]
  Constant2 : Constant  Value=[0 0 1]
  Dot Product : DotProduct  OutDataTypeStr=Inherit: Inherit via internal rule
  Dot Product1 : DotProduct  OutDataTypeStr=Inherit: Inherit via internal rule
  Dot Product2 : DotProduct  OutDataTypeStr=Inherit: Inherit via internal rule
  Gain1 : Gain  Gain=180/pi
  Gain3 : Gain  Gain=180/pi
  Gain4 : Gain  Gain=180/pi
  Math Function1 : Math  Operator=transpose  SignedPower=on
  Mux : Mux  Inputs=3
  Normalize Vector1 : vrlib/Utilities/Normalize Vector  maxzero=0
  Normalize Vector2 : vrlib/Utilities/Normalize Vector  maxzero=0
  Normalize Vector3 : vrlib/Utilities/Normalize Vector  maxzero=0
  Trigonometric Function : Trigonometry  Operator=acos
  Trigonometric Function1 : Trigonometry  Operator=acos
  Trigonometric Function2 : Trigonometry  Operator=acos
  product 1 : Product  Multiplication=Matrix(*)  RndMeth=Zero
  product 2 : Product  Multiplication=Matrix(*)  RndMeth=Zero
  product 3 : Product  Multiplication=Matrix(*)  RndMeth=Zero
  Cone Angles : Outport
  wires:
  product 1/1 -> Normalize Vector1/1
  Reference Vector/1 -> Dot Product/1, Dot Product1/1, Dot Product2/1
  Normalize Vector1/1 -> Dot Product/2
  Dot Product/1 -> Trigonometric Function/1
  Trigonometric Function/1 -> Gain1/1
  Attitude/1 -> Math Function1/1
  Constant/1 -> product 1/2
  Math Function1/1 -> product 1/1, product 2/1, product 3/1
  Mux/1 -> Cone Angles/1
  Gain1/1 -> Mux/1
  Dot Product1/1 -> Trigonometric Function1/1
  Trigonometric Function1/1 -> Gain3/1
  Dot Product2/1 -> Trigonometric Function2/1
  Trigonometric Function2/1 -> Gain4/1
  Gain3/1 -> Mux/2
  Gain4/1 -> Mux/3
  product 2/1 -> Normalize Vector2/1
  Constant1/1 -> product 2/2
  product 3/1 -> Normalize Vector3/1
  Constant2/1 -> product 3/2
  Normalize Vector2/1 -> Dot Product1/2
  Normalize Vector3/1 -> Dot Product2/2

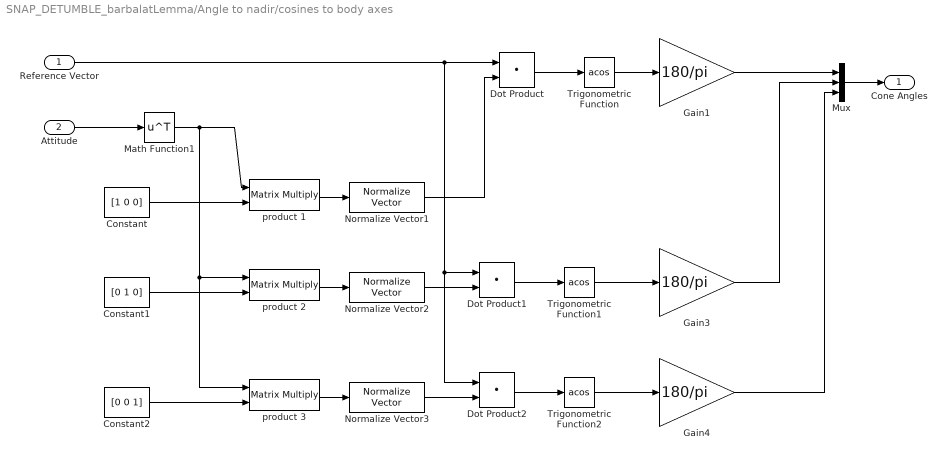
== system SNAP_DETUMBLE_barbalatLemma/Angle to nadir/cosines to body axes ==
  Reference Vector : Inport
  Attitude : Inport  Port=2
  Constant : Constant  Value=[1 0 0]
  Constant1 : Constant  Value=[0 1 0]
  Constant2 : Constant  Value=[0 0 1]
  Dot Product : DotProduct  OutDataTypeStr=Inherit: Inherit via internal rule
  Dot Product1 : DotProduct  OutDataTypeStr=Inherit: Inherit via internal rule
  Dot Product2 : DotProduct  OutDataTypeStr=Inherit: Inherit via internal rule
  Gain1 : Gain  Gain=180/pi
  Gain3 : Gain  Gain=180/pi
  Gain4 : Gain  Gain=180/pi
  Math Function1 : Math  Operator=transpose  SignedPower=on
  Mux : Mux  Inputs=3
  Normalize Vector1 : vrlib/Utilities/Normalize Vector  maxzero=0
  Normalize Vector2 : vrlib/Utilities/Normalize Vector  maxzero=0
  Normalize Vector3 : vrlib/Utilities/Normalize Vector  maxzero=0
  Trigonometric Function : Trigonometry  Operator=acos
  Trigonometric Function1 : Trigonometry  Operator=acos
  Trigonometric Function2 : Trigonometry  Operator=acos
  product 1 : Product  Multiplication=Matrix(*)  RndMeth=Zero
  product 2 : Product  Multiplication=Matrix(*)  RndMeth=Zero
  product 3 : Product  Multiplication=Matrix(*)  RndMeth=Zero
  Cone Angles : Outport
  wires:
  product 1/1 -> Normalize Vector1/1
  Reference Vector/1 -> Dot Product/1, Dot Product1/1, Dot Product2/1
  Normalize Vector1/1 -> Dot Product/2
  Dot Product/1 -> Trigonometric Function/1
  Trigonometric Function/1 -> Gain1/1
  Attitude/1 -> Math Function1/1
  Constant/1 -> product 1/2
  Math Function1/1 -> product 1/1, product 2/1, product 3/1
  Mux/1 -> Cone Angles/1
  Gain1/1 -> Mux/1
  Dot Product1/1 -> Trigonometric Function1/1
  Trigonometric Function1/1 -> Gain3/1
  Dot Product2/1 -> Trigonometric Function2/1
  Trigonometric Function2/1 -> Gain4/1
  Gain3/1 -> Mux/2
  Gain4/1 -> Mux/3
  product 2/1 -> Normalize Vector2/1
  Constant1/1 -> product 2/2
  product 3/1 -> Normalize Vector3/1
  Constant2/1 -> product 3/2
  Normalize Vector2/1 -> Dot Product1/2
  Normalize Vector3/1 -> Dot Product2/2

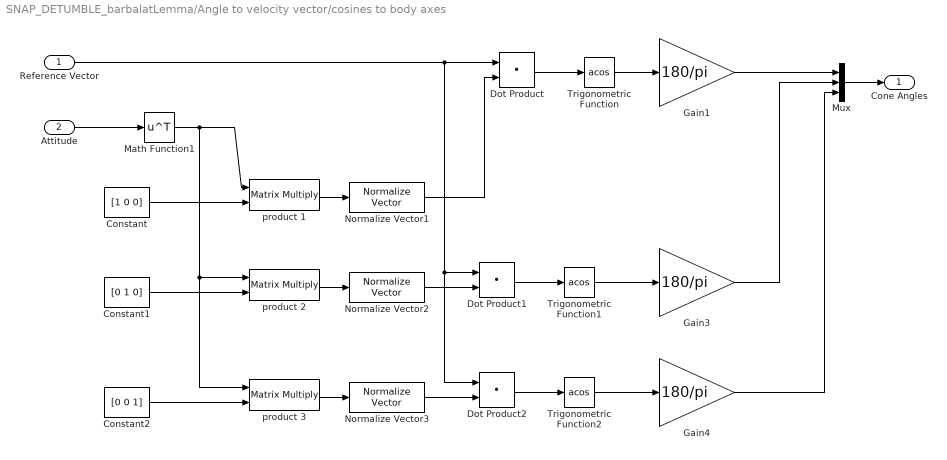
== system SNAP_DETUMBLE_barbalatLemma/Angle to velocity vector/cosines to body axes ==
  Reference Vector : Inport
  Attitude : Inport  Port=2
  Constant : Constant  Value=[1 0 0]
  Constant1 : Constant  Value=[0 1 0]
  Constant2 : Constant  Value=[0 0 1]
  Dot Product : DotProduct  OutDataTypeStr=Inherit: Inherit via internal rule
  Dot Product1 : DotProduct  OutDataTypeStr=Inherit: Inherit via internal rule
  Dot Product2 : DotProduct  OutDataTypeStr=Inherit: Inherit via internal rule
  Gain1 : Gain  Gain=180/pi
  Gain3 : Gain  Gain=180/pi
  Gain4 : Gain  Gain=180/pi
  Math Function1 : Math  Operator=transpose  SignedPower=on
  Mux : Mux  Inputs=3
  Normalize Vector1 : vrlib/Utilities/Normalize Vector  maxzero=0
  Normalize Vector2 : vrlib/Utilities/Normalize Vector  maxzero=0
  Normalize Vector3 : vrlib/Utilities/Normalize Vector  maxzero=0
  Trigonometric Function : Trigonometry  Operator=acos
  Trigonometric Function1 : Trigonometry  Operator=acos
  Trigonometric Function2 : Trigonometry  Operator=acos
  product 1 : Product  Multiplication=Matrix(*)  RndMeth=Zero
  product 2 : Product  Multiplication=Matrix(*)  RndMeth=Zero
  product 3 : Product  Multiplication=Matrix(*)  RndMeth=Zero
  Cone Angles : Outport
  wires:
  product 1/1 -> Normalize Vector1/1
  Reference Vector/1 -> Dot Product/1, Dot Product1/1, Dot Product2/1
  Normalize Vector1/1 -> Dot Product/2
  Dot Product/1 -> Trigonometric Function/1
  Trigonometric Function/1 -> Gain1/1
  Attitude/1 -> Math Function1/1
  Constant/1 -> product 1/2
  Math Function1/1 -> product 1/1, product 2/1, product 3/1
  Mux/1 -> Cone Angles/1
  Gain1/1 -> Mux/1
  Dot Product1/1 -> Trigonometric Function1/1
  Trigonometric Function1/1 -> Gain3/1
  Dot Product2/1 -> Trigonometric Function2/1
  Trigonometric Function2/1 -> Gain4/1
  Gain3/1 -> Mux/2
  Gain4/1 -> Mux/3
  product 2/1 -> Normalize Vector2/1
  Constant1/1 -> product 2/2
  product 3/1 -> Normalize Vector3/1
  Constant2/1 -> product 3/2
  Normalize Vector2/1 -> Dot Product1/2
  Normalize Vector3/1 -> Dot Product2/2

== system SNAP_DETUMBLE_barbalatLemma/ECI2ECEF - position/Direction Cosine Matrix ECI to ECEF1 ==
  JD : Inport  OutMin=0  PortDimensions=1
  AddParam : Constant  Value="[0  0]"
  Common Time Calculation : Subsystem
  IAUReduction : Subsystem  AncestorBlock=aerolibtransform2sys/IAU20002006  mask{deltaT=Sec, Sdata=0, XYdata=0}
      mask prompts: deltaT "Time Increment"
      mask init:
      | load aeroCIP2006.mat
      mask TypeOptions deltaT: None | Day | Hour | Min | Sec
  PolarMotion : Constant  Value="[0  0]"
  deltaAT : Constant  Value=[0]
  deltaUT1 : Constant  Value=[0]
  DCM : Outport
  wires:
  deltaAT/1 -> Common Time Calculation/3(deltaAT)
  deltaUT1/1 -> Common Time Calculation/2(deltaUT1)
  PolarMotion/1 -> IAUReduction/6("[xp,yp]")
  Common Time Calculation/3(jdTT) -> IAUReduction/5(jdTT)
  AddParam/1 -> IAUReduction/1("[dX,dY]")
  Common Time Calculation/1(tTT) -> IAUReduction/3(tTT)
  Common Time Calculation/2(ssUT) -> IAUReduction/4(ssUT)
  IAUReduction/1(DCM) -> DCM/1
  JD/1 -> IAUReduction/2("JD "), Common Time Calculation/1(JD)

== system SNAP_DETUMBLE_barbalatLemma/Hysteresis Material/Eearth L-Shell Magnetic Model ==
  note: B(R) = ( a^3 * H0 / R^3 ) * [ 3(m.R)R-m ]
  note: Mag field at X, in ECEF
  note: mag field in ECI (Tesla)
  Position in ECI : Inport
  Constant3 : Constant  Value=3
  Divide1 : Product  Inputs=*/
  Dot Product : DotProduct  OutDataTypeStr=Inherit: Inherit via internal rule
  Dot Product - magnitude squared : DotProduct  OutDataTypeStr=Inherit: Inherit via internal rule
  ECEF2ECI : Subsystem
  ECI2ECEF - position1 : Subsystem
  Gain : Gain  Gain=3
  Gain1 : Gain  Gain=SNAP_CONST_a3H0
  Math Cubing : Math  Operator=pow  SignedPower=on
  Normalize Vector : vrlib/Utilities/Normalize Vector  maxzero=0
  Product1 : Product  RndMeth=Zero
  Sum1 : Sum  Inputs=|-+
  "m (unit vector, magnetic dipole in ECEF)" : Constant  Value=SNAP_CONST_earth_mag_dipole
  sqrt : Math  Operator=sqrt  SignedPower=on
  B (Tesla) in ECI : Outport
  wires:
  "m (unit vector, magnetic dipole in ECEF)"/1 -> Dot Product/1, Sum1/1
  ECI2ECEF - position1/1(ECEF) -> Dot Product - magnitude squared/2, Dot Product - magnitude squared/1, Normalize Vector/1
  Dot Product/1 -> Product1/1
  Product1/1 -> Gain/1
  Gain/1 -> Sum1/2
  Sum1/1 -> Gain1/1
  Gain1/1 -> Divide1/1
  Dot Product - magnitude squared/1 -> sqrt/1
  sqrt/1 -> Math Cubing/1
  Constant3/1 -> Math Cubing/2
  Math Cubing/1 -> Divide1/2
  Divide1/1 -> ECEF2ECI/1(ECEF)
  Normalize Vector/1 -> Dot Product/2, Product1/2
  ECEF2ECI/1(ECI) -> B (Tesla) in ECI/1
  Position in ECI/1 -> ECI2ECEF - position1/1(ECI)

== system SNAP_DETUMBLE_barbalatLemma/Hysteresis Material/Hysteresis Curve Model ==
  H : Inport
  Constant1 : Constant  Value=SNAP_Bs* 1e4
  Constant2 : Constant  Value=SNAP_Br* 1e4
  Constant3 : Constant  Value=SNAP_Hc
  Derivative : Derivative
  Gain : Gain  Gain=10000
  Gain2 : Gain  Gain=1/10000
  Hysteresis Model : MATLAB Function  TreatAsAtomicUnit=on
  Integrator : Integrator  InitialCondition=10000
  Rate Transition : RateTransition  Deterministic=off  OutPortSampleTimeOpt=Inherit  OutPortSampleTime=0.05
  Saturation1 : Saturate  UpperLimit=SNAP_Bs  LowerLimit=-SNAP_Bs
  B : Outport
  wires:
  Hysteresis Model/1(DBDT) -> Integrator/1
  Integrator/1 -> Gain2/1
  Gain/1 -> Hysteresis Model/1(B)
  Gain2/1 -> Saturation1/1
  Saturation1/1 -> Gain/1, B/1
  Rate Transition/1 -> Derivative/1, Hysteresis Model/2(H)
  Derivative/1 -> Hysteresis Model/3(DHDT)
  H/1 -> Rate Transition/1
  Constant1/1 -> Hysteresis Model/4(Bsx)
  Constant2/1 -> Hysteresis Model/5(Brx)
  Constant3/1 -> Hysteresis Model/6(Hcx)

== system SNAP_DETUMBLE_barbalatLemma/MAGNETORQUER MODEL/x-axis ==
  I_desired_b : Inport
  Abs2 : Abs
  Constant1 : Constant  Value=boira_Imax(1)
  Divide : Product  Inputs=*/
  Non-linearity : Lookup_n-D  NumberOfTableDimensions=1  BreakpointsForDimension1=lookup_breakpoints_mtorquer  Table=lookup_tabledata_mtorquer  InternalRulePriority=Speed  RndMeth=Simplest
  PWM2 : simulink/Discontinuities/PWM  DisableCoverage=on  Period=0.1  InitialDelay=0  DisallowZeroDutyCycle=off  RunAtFixedTimeIntervals=on  SampleTime=0.02
  Product2 : Product  Inputs=3
  Saturation1 : Saturate  UpperLimit=boira_Imax(1)  LowerLimit=-boira_Imax(1)
  Sign : Signum
  I_obtained_b : Outport
  wires:
  I_desired_b/1 -> Saturation1/1
  Saturation1/1 -> Sign/1, Abs2/1
  Abs2/1 -> Divide/1
  Divide/1 -> PWM2/1
  Constant1/1 -> Non-linearity/1, Divide/2
  PWM2/1 -> Product2/1
  Sign/1 -> Product2/2
  Non-linearity/1 -> Product2/3
  Product2/1 -> I_obtained_b/1

== system SNAP_DETUMBLE_barbalatLemma/MAGNETORQUER MODEL/y-axis ==
  I_desired_b : Inport
  Abs2 : Abs
  Constant1 : Constant  Value=boira_Imax(2)
  Divide : Product  Inputs=*/
  Non-linearity : Lookup_n-D  NumberOfTableDimensions=1  BreakpointsForDimension1=lookup_breakpoints_mtorquer  Table=lookup_tabledata_mtorquer  InternalRulePriority=Speed  RndMeth=Simplest
  PWM2 : simulink/Discontinuities/PWM  DisableCoverage=on  Period=0.1  InitialDelay=0  DisallowZeroDutyCycle=off  RunAtFixedTimeIntervals=on  SampleTime=0.02
  Product2 : Product  Inputs=3
  Saturation1 : Saturate  UpperLimit=boira_Imax(2)  LowerLimit=-boira_Imax(2)
  Sign : Signum
  I_obtained_b : Outport
  wires:
  I_desired_b/1 -> Saturation1/1
  Saturation1/1 -> Sign/1, Abs2/1
  Abs2/1 -> Divide/1
  Divide/1 -> PWM2/1
  Constant1/1 -> Non-linearity/1, Divide/2
  PWM2/1 -> Product2/1
  Sign/1 -> Product2/2
  Non-linearity/1 -> Product2/3
  Product2/1 -> I_obtained_b/1

== system SNAP_DETUMBLE_barbalatLemma/MAGNETORQUER MODEL/z-axis ==
  I_desired_b : Inport
  Abs2 : Abs
  Constant1 : Constant  Value=boira_Imax(3)
  Divide : Product  Inputs=*/
  Non-linearity : Lookup_n-D  NumberOfTableDimensions=1  BreakpointsForDimension1=lookup_breakpoints_mtorquer  Table=lookup_tabledata_mtorquer  InternalRulePriority=Speed  RndMeth=Simplest
  PWM2 : simulink/Discontinuities/PWM  DisableCoverage=on  Period=0.1  InitialDelay=0  DisallowZeroDutyCycle=off  RunAtFixedTimeIntervals=on  SampleTime=0.02
  Product2 : Product  Inputs=3
  Saturation1 : Saturate  UpperLimit=boira_Imax(3)  LowerLimit=-boira_Imax(3)
  Sign : Signum
  I_obtained_b : Outport
  wires:
  I_desired_b/1 -> Saturation1/1
  Saturation1/1 -> Sign/1, Abs2/1
  Abs2/1 -> Divide/1
  Divide/1 -> PWM2/1
  Constant1/1 -> Non-linearity/1, Divide/2
  PWM2/1 -> Product2/1
  Sign/1 -> Product2/2
  Non-linearity/1 -> Product2/3
  Product2/1 -> I_obtained_b/1

== system SNAP_DETUMBLE_barbalatLemma/Magnets/Eearth L-Shell Magnetic Model ==
  note: B(R) = ( a^3 * H0 / R^3 ) * [ 3(m.R)R-m ]
  note: Mag field at X, in ECEF
  note: mag field in ECI (Tesla)
  Position in ECI : Inport
  Constant3 : Constant  Value=3
  Divide1 : Product  Inputs=*/
  Dot Product : DotProduct  OutDataTypeStr=Inherit: Inherit via internal rule
  Dot Product - magnitude squared : DotProduct  OutDataTypeStr=Inherit: Inherit via internal rule
  ECEF2ECI : Subsystem
  ECI2ECEF - position1 : Subsystem
  Gain : Gain  Gain=3
  Gain1 : Gain  Gain=SNAP_CONST_a3H0
  Math Cubing : Math  Operator=pow  SignedPower=on
  Normalize Vector : vrlib/Utilities/Normalize Vector  maxzero=0
  Product1 : Product  RndMeth=Zero
  Sum1 : Sum  Inputs=|-+
  "m (unit vector, magnetic dipole in ECEF)" : Constant  Value=SNAP_CONST_earth_mag_dipole
  sqrt : Math  Operator=sqrt  SignedPower=on
  B (Tesla) in ECI : Outport
  wires:
  "m (unit vector, magnetic dipole in ECEF)"/1 -> Dot Product/1, Sum1/1
  ECI2ECEF - position1/1(ECEF) -> Dot Product - magnitude squared/2, Dot Product - magnitude squared/1, Normalize Vector/1
  Dot Product/1 -> Product1/1
  Product1/1 -> Gain/1
  Gain/1 -> Sum1/2
  Sum1/1 -> Gain1/1
  Gain1/1 -> Divide1/1
  Dot Product - magnitude squared/1 -> sqrt/1
  sqrt/1 -> Math Cubing/1
  Constant3/1 -> Math Cubing/2
  Math Cubing/1 -> Divide1/2
  Divide1/1 -> ECEF2ECI/1(ECEF)
  Normalize Vector/1 -> Dot Product/2, Product1/2
  ECEF2ECI/1(ECI) -> B (Tesla) in ECI/1
  Position in ECI/1 -> ECI2ECEF - position1/1(ECI)

== system SNAP_DETUMBLE_barbalatLemma/ECI2ECEF - position/Direction Cosine Matrix ECI to ECEF1/Common Time Calculation ==
  JD : Inport
  deltaUT1 : Inport  Port=2
  deltaAT : Inport  Port=3
  Bias : Bias  Bias=32.184  SaturateOnIntegerOverflow=off
  Bias1 : Bias  Bias=-51544.5  SaturateOnIntegerOverflow=off
  Gain : Gain  Gain=1/36525
  Sum2 : Sum  Inputs=|++
  secGain : Gain  Gain=1/86400
  tTT : Outport
  ssUT : Outport  Port=2
  jdTT : Outport  Port=3
  wires:
  deltaAT/1 -> Bias/1
  Bias/1 -> secGain/1
  Bias1/1 -> Gain/1
  Gain/1 -> tTT/1
  deltaUT1/1 -> ssUT/1
  secGain/1 -> Sum2/2
  JD/1 -> Sum2/1
  Sum2/1 -> Bias1/1, jdTT/1

== system SNAP_DETUMBLE_barbalatLemma/ECI2ECEF - position/Direction Cosine Matrix ECI to ECEF1/IAUReduction ==
  "[dX,dY]" : Inport
  "JD " : Inport  Port=2
  tTT : Inport  Port=3
  ssUT : Inport  Port=4
  jdTT : Inport  Port=5
  "[xp,yp]" : Inport  Port=6
  Additional Time Calculations : Subsystem
  Celestial motion of the CIP : Subsystem
  Earth Rotation : Subsystem
  Polar Motion : Subsystem
  Product : Product  Inputs=3  Multiplication=Matrix(*)
  Terminator : Terminator
  tTT1 : InportShadow  Port=3
  DCM : Outport
  wires:
  "[xp,yp]"/1 -> Polar Motion/2("[xp,yp]")
  Polar Motion/1(W) -> Product/1
  Celestial motion of the CIP/1(Q) -> Product/3
  jdTT/1 -> Terminator/1
  Product/1 -> DCM/1
  ssUT/1 -> Additional Time Calculations/1(ssUT)
  "JD "/1 -> Additional Time Calculations/2("JD ")
  tTT/1 -> Celestial motion of the CIP/2(tTT)
  "[dX,dY]"/1 -> Celestial motion of the CIP/1("[dX,dY]")
  Earth Rotation/1(R) -> Product/2
  tTT1/1 -> Polar Motion/1(tTT)
  Additional Time Calculations/1(jdElapsed) -> Earth Rotation/1(jdElapsed)
  Additional Time Calculations/2(jdFraction) -> Earth Rotation/2(jdFraction)

== system SNAP_DETUMBLE_barbalatLemma/Hysteresis Material/Eearth L-Shell Magnetic Model/ECEF2ECI ==
  ECEF : Inport
  Constant1 : Constant  Value=[0 0]
  Constant3 : Constant  Value=SNAP_starting_ECI2ECEF_dcm
  Gain1 : Gain  Gain=-1
  Math Function2 : Math  Operator=transpose  SignedPower=on
  Mux1 : Mux  Inputs=2
  Ramp2 : simulink/Sources/Ramp  slope="7.292115856e-5   %2*pi/(24*60*60)  %radians/second (one rotation per day )"  start=0  InitialOutput=0
  Rotation Angles to Direction Cosine Matrix1 : sharedtransform/Rotation Angles to Direction Cosine Matrix  rotationOrder=ZYX  aMode=aMode
  product 2 : Product  Multiplication=Matrix(*)  RndMeth=Zero
  product 4 : Product  Multiplication=Matrix(*)  RndMeth=Zero
  ECI : Outport
  wires:
  ECEF/1 -> product 4/1
  Ramp2/1 -> Gain1/1
  Gain1/1 -> Mux1/1
  Mux1/1 -> Rotation Angles to Direction Cosine Matrix1/1
  Constant1/1 -> Mux1/2
  product 2/1 -> Math Function2/1
  Rotation Angles to Direction Cosine Matrix1/1 -> product 2/2
  Constant3/1 -> product 2/1
  Math Function2/1 -> product 4/2
  product 4/1 -> ECI/1
